simulink model "task_3"  (R2023a)
settings: Solver=VariableStepAuto  StartTime=0.0  StopTime=10.0  RelTol=1e-8
settings Model: Creator=user  LastModifiedBy=user

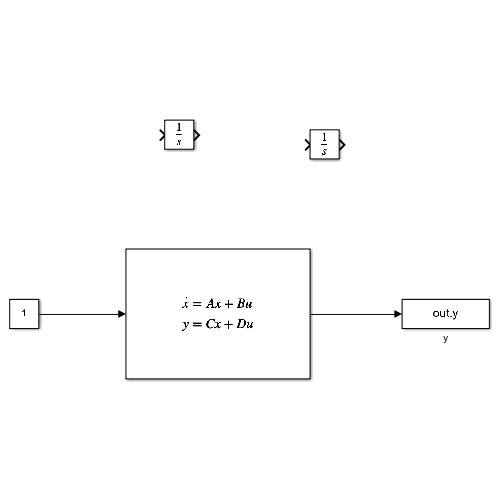
[thumbnail: Simulink's stored preview of the top-level diagram]
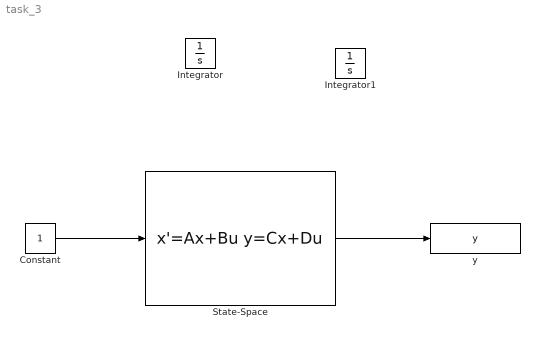
== system task_3 ==
  Constant : Constant
  Integrator : Integrator
  Integrator1 : Integrator
  State-Space : StateSpace  A=|  B="[0;  0;  0;  0]"  C="[0  1  0  1]"  D=[0]  InitialCondition=[0; 1; -1; 0]  ParameterTunability=Unconstrained
      | [0  3  0  0; -3  0  0  0;  0  0  -5  7;
      |     0  0  -7  -5]
  y : ToWorkspace  VariableName=y  SaveFormat=Timeseries  SampleTime=-1
  wires:
  Constant/1 -> State-Space/1
  State-Space/1 -> y/1
